simulink model "complex_fir_core"  (R2013a)
settings: Solver=VariableStepDiscrete  SolverMode=SingleTasking  StartTime=0.0  StopTime=2000  RelTol=1e-3
undefined symbols (not defined in the file or in its folder): pfb_coeff_gen_calc
libraries: xbsIndex_r4 x1618, casper_library_misc x112
(part 1 of 19)
settings Model: Creator=rprimian  LastModifiedBy=jack
settings Model: ModifiedComment=|
  | jack -- Wed Mar 18 10:34:12 2015 -- Version 1.45
  | resynth -lc off -equiv_reg_removal no
settings Model: ModifiedHistory=|
  | jack -- Wed Mar 18 10:34:12 2015 -- Version 1.45
  | resynth -lc off -equiv_reg_removal no
  | 
  | jack -- Wed Mar 18 10:28:24 2015 -- Version 1.44
  | change sync fanouter to have latency of 4 (max fanout 2)
  | 
  | jack -- Sun Jan 11 19:12:21 2015 -- Version 1.43
  | redrew with sync_delays implemented in srls when delay < 1024 (basically, always)
  | 
  | jack -- Sat Jan 10 15:01:06 2015 -- Version 1.42
  | generated
  | 
  | jack -- Sat Jan 10 13:10:56 2015 -- Version 1.41
  | update draw script to pipeline both fir cast blocks (was only pipelineing real one)
  | 
  | jack -- Fri Jan 09 11:30:49 2015 -- Version 1.40
  | 
  | 
  | jack -- Fri Jan 09 10:35:18 2015 -- Version 1.39
  | change add latency to 2. xlupdate model to 14.7
  | 
  | jack -- Fri Dec 05 12:22:04 2014 -- Version 1.38
  | compile test
  | 
  | cast latency3
settings DataIOCC: SignalLoggingSaveFormat=ModelDataLogs
settings OptimizationCC: InlineParams=on  ExpressionDepthLimit=2147483647
settings DebuggingCC: FcnCallInpInsideContextMsg=UseLocalSettings
settings GRTTargetCC: CombineOutputUpdateFcns=off  GRTInterface=on

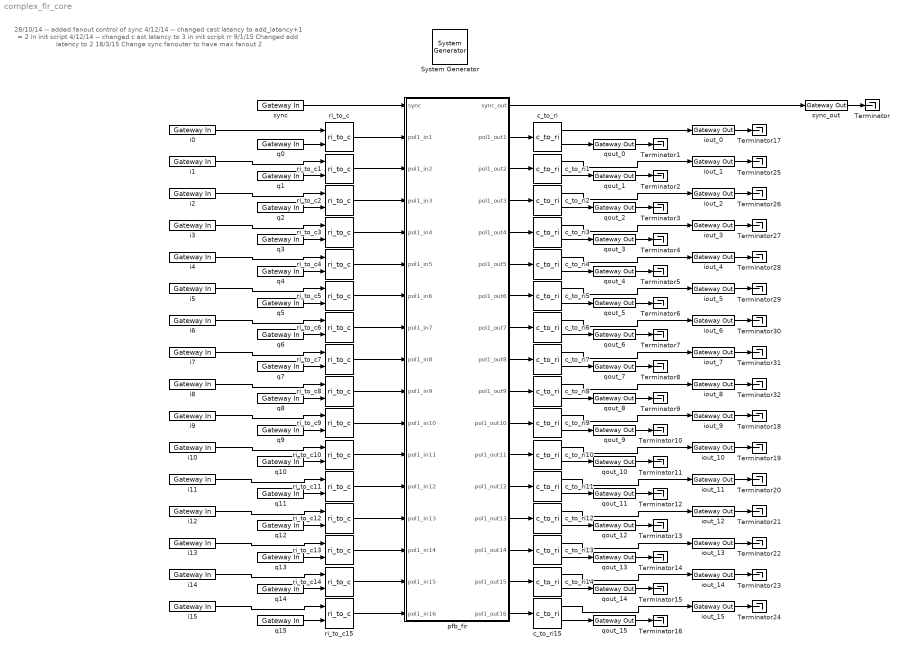
== system complex_fir_core ==
  note: 28/10/14 -- added fanout control of sync
      | 4/12/14 -- changed cast latency to add_latency+1 = 2 in init script
      | 4/12/14 -- changed c ast latency to 3 in init script rr
      | 9/1/15 Changed add latency to 2
      | 18/3/15 Change sync fanouter to have max fanout 2
  " System Generator" : xbsIndex_r4/ System Generator  Tag=genX  xilinxfamily=virtex6  part=xc6vsx475t  speed=-1  package=ff1759  synthesis_tool=XST  clock_wrapper=Clock Enables  directory=./complex_fir_core  proj_type=Project Navigator  Synth_file=XST Defaults  Impl_file=ISE Defaults  testbench=off  simulink_period=1  sysclk_period=3  dcm_input_clock_period=100  incr_netlist=off  trim_vbits=Everywhere in SubSystem  dbl_ovrd=According to Block Masks  core_generation=According to Block Masks  run_coregen=off  deprecated_control=off  eval_field=0  block_type=sysgen
      settings: block_version=11.4
  Terminator{,1..32} (33 alike) : Terminator
  c_to_ri{,1..15} (16 alike) : casper_library_misc/c_to_ri  n_bits=18  bin_pt=17
  i{0..15} (16 alike) : xbsIndex_r4/Gateway In  gui_display_data_type=Fixed-point  arith_type="Signed  (2's comp)"  n_bits=8  bin_pt=7  preci_type=Single  exp_width=8  frac_width=24  quantization="Round  (unbiased: +/- Inf)"  overflow=Saturate  period=1  dbl_ovrd=off  timing_constraint=None  locs_specified=off  LOCs={}  UseAsADC=off  ADCChannel='1'  inherit_from_input=off  hdl_port=on  block_type=gatewayin
      settings: infoedit="Gateway in block.  Converts inputs of type Simulink integer, double and fixed point to  Xilinx fixed point type.<br><br>Hardware notes:  In hardware these blocks become top level input ports."  block_version=11.4
  iout_{0..15} (16 alike) : xbsIndex_r4/Gateway Out  inherit_from_input=off  hdl_port=on  timing_constraint=None  locs_specified=off  LOCs={}  UseAsDAC=off  DACChannel='1'  block_type=gatewayout
      settings: infoedit="Gateway out block.  Converts Xilinx fixed point inputs into ouputs of type Simulink integer, double, or fixed point.<br><br>Hardware notes:  In hardware these blocks become top level output ports or are discarded, depending on how they are configured."  block_version=11.4
  pfb_fir : Subsystem  Tag=casper:pfb_fir  AncestorBlock=casper_library_pfbs/pfb_fir  mask(pfb_fir){PFBSize=12, TotalTaps=4, WindowType=hamming, n_inputs=4, MakeBiplex=off, BitWidthIn=8, BitWidthOut=18, CoeffBitWidth=18, CoeffDistMem=off, add_latency=2, mult_latency=3, bram_latency=3, fan_latency=1, quantization=Round  (unbiased: +/- Inf), fwidth=1, mult_spec=1, coeffs_share=on}
      mask prompts: PFBSize "Size of PFB: (2^? pnts)"; TotalTaps "Total Number of Taps:"; WindowType "Windowing Function:"; n_inputs "Number of Simultaneous Inputs: (2^?)"; MakeBiplex "Make Biplex?"; BitWidthIn "Input Bitwidth:"; BitWidthOut "Output Bitwidth:"; CoeffBitWidth "Coefficient Bitwidth:"; CoeffDistMem "Use Distributed Memory for Coeffs"; add_latency "Add Latency"; mult_latency "Mult Latency"; bram_latency "BRAM Latency"; fan_latency "Fanout Latency"; quantization "Quantization Behavior"; fwidth "Bin Width Scaling (normal=1)"; mult_spec "Multiplier specification (0=core, 1=embedded, 2=behavioural) (left=1st tap, or just one value)"; coeffs_share "Share coefficients between polarisations (use less BRAM)?"
      mask init:
      | pfb_fir_init(gcb, ...
      |     'PFBSize', PFBSize, ...
      |     'TotalTaps', TotalTaps, ...
      |     'WindowType', WindowType, ...
      |     'n_inputs', n_inputs, ...
      |     'MakeBiplex', MakeBiplex, ...
      |     'BitWidthIn', BitWidthIn, ...
      |     'BitWidthOut', BitWidthOut, ...
      |     'CoeffBitWidth', CoeffBitWidth, ...
      |     'CoeffDistMem', CoeffDistMem, ...
      |     'add_latency', add_latency, ...
      |     'mult_latency', mult_latency, ...
      |     'bram_latency', bram_latency, ...
      |     'fan_latency', fan_latency, ...
      |     'quantization', quantization, ...
      |     'fwidth', fwidth, ...
      |     'mult_spec', mult_spec, ...
      |     'coeffs_share', coeffs_share);
      settings: AttributesFormatString=|
      | taps=4, add_latency=2
      | max scale 0.596
      mask Help: eval('xlWeb(''http://casper.berkeley.edu/wiki/Pfb_fir'')')
      mask Callback TotalTaps:
      | %num_taps = eval(get_param(gcb, 'TotalTaps'));
      | %old_vec = eval(get_param(gcb, 'mult_spec'));
      | 
      | %vec = 2.*ones(1,num_taps);
      | %old_size = length(old_vec);
      | 
      | %if(old_size <= num_taps),
      | %   new_size = old_size;
      | %else,
      | %    new_size = num_taps;
      | %end
      | 
      | %for n = 1:new_size, vec(n) = old_vec(n); end
      | %set_param(gcb, 'mult_spec', mat2str(vec));
      mask TypeOptions WindowType: bartlett | barthannwin | blackman | blackmanharris | bohamwin | chebwin | flattopwin | gausswin | hamming | hann | kaiser | nuttallwin | parzenwin | rectwin | tukeywin | triang | userwindow
      mask TypeOptions quantization: Truncate | Round  (unbiased: +/- Inf) | Round  (unbiased: Even Values)
      mask Callback fwidth:
      | %num_taps = eval(get_param(gcb, 'TotalTaps'));
      | %old_vec = eval(get_param(gcb, 'mult_spec'));
      | 
      | %vec = 2.*ones(1,num_taps);
      | %old_size = length(old_vec);
      | 
      | %if(old_size <= num_taps),
      | %    new_size = old_size;
      | %else,
      | %    new_size = num_taps;
      | %end
      | 
      | %for n = 1:new_size, vec(n) = old_vec(n); end
      | %set_param(gcb, 'mult_spec', mat2str(vec));
      mask Callback mult_spec:
      | %num_taps = eval(get_param(gcb, 'TotalTaps'));
      | %old_vec = eval(get_param(gcb, 'mult_spec'));
      | 
      | %vec = 2.*ones(1,num_taps);
      | %old_size = length(old_vec);
      | 
      | %if(old_size <= num_taps),
      | %    new_size = old_size;
      | %else,
      | %    new_size = num_taps;
      | %end
      | 
      | %for n = 1:new_size, vec(n) = old_vec(n); end
      | %set_param(gcb, 'mult_spec', mat2str(vec));
  q{0..15} (16 alike) : xbsIndex_r4/Gateway In  gui_display_data_type=Fixed-point  arith_type="Signed  (2's comp)"  n_bits=8  bin_pt=7  preci_type=Single  exp_width=8  frac_width=24  quantization="Round  (unbiased: +/- Inf)"  overflow=Saturate  period=1  dbl_ovrd=off  timing_constraint=None  locs_specified=off  LOCs={}  UseAsADC=off  ADCChannel='1'  inherit_from_input=off  hdl_port=on  block_type=gatewayin
      settings: infoedit="Gateway in block.  Converts inputs of type Simulink integer, double and fixed point to  Xilinx fixed point type.<br><br>Hardware notes:  In hardware these blocks become top level input ports."  block_version=11.4
  qout_{0..15} (16 alike) : xbsIndex_r4/Gateway Out  inherit_from_input=off  hdl_port=on  timing_constraint=None  locs_specified=off  LOCs={}  UseAsDAC=off  DACChannel='1'  block_type=gatewayout
      settings: infoedit="Gateway out block.  Converts Xilinx fixed point inputs into ouputs of type Simulink integer, double, or fixed point.<br><br>Hardware notes:  In hardware these blocks become top level output ports or are discarded, depending on how they are configured."  block_version=11.4
  ri_to_c{,1..15} (16 alike) : casper_library_misc/ri_to_c
  sync : xbsIndex_r4/Gateway In  gui_display_data_type=Fixed-point  arith_type=Boolean  n_bits=1  bin_pt=0  preci_type=Single  exp_width=8  frac_width=24  quantization="Round  (unbiased: +/- Inf)"  overflow=Saturate  period=1  dbl_ovrd=off  timing_constraint=None  locs_specified=off  LOCs={}  UseAsADC=off  ADCChannel='1'  inherit_from_input=off  hdl_port=on  block_type=gatewayin
      settings: infoedit="Gateway in block.  Converts inputs of type Simulink integer, double and fixed point to  Xilinx fixed point type.<br><br>Hardware notes:  In hardware these blocks become top level input ports."  block_version=11.4
  sync_out : xbsIndex_r4/Gateway Out  inherit_from_input=off  hdl_port=on  timing_constraint=None  locs_specified=off  LOCs={}  UseAsDAC=off  DACChannel='1'  block_type=gatewayout
      settings: infoedit="Gateway out block.  Converts Xilinx fixed point inputs into ouputs of type Simulink integer, double, or fixed point.<br><br>Hardware notes:  In hardware these blocks become top level output ports or are discarded, depending on how they are configured."  block_version=11.4
  wires:
  sync_out/1 -> Terminator/1
  qout_0/1 -> Terminator1/1
  qout_1/1 -> Terminator2/1
  qout_2/1 -> Terminator3/1
  qout_3/1 -> Terminator4/1
  qout_4/1 -> Terminator5/1
  qout_5/1 -> Terminator6/1
  qout_6/1 -> Terminator7/1
  qout_7/1 -> Terminator8/1
  qout_8/1 -> Terminator9/1
  qout_9/1 -> Terminator10/1
  qout_10/1 -> Terminator11/1
  qout_11/1 -> Terminator12/1
  qout_12/1 -> Terminator13/1
  qout_13/1 -> Terminator14/1
  qout_14/1 -> Terminator15/1
  qout_15/1 -> Terminator16/1
  ri_to_c/1 -> pfb_fir/2(pol1_in1)
  ri_to_c1/1 -> pfb_fir/3(pol1_in2)
  sync/1 -> pfb_fir/1(sync)
  ri_to_c2/1 -> pfb_fir/4(pol1_in3)
  ri_to_c3/1 -> pfb_fir/5(pol1_in4)
  ri_to_c5/1 -> pfb_fir/7(pol1_in6)
  ri_to_c4/1 -> pfb_fir/6(pol1_in5)
  ri_to_c7/1 -> pfb_fir/9(pol1_in8)
  ri_to_c6/1 -> pfb_fir/8(pol1_in7)
  ri_to_c10/1 -> pfb_fir/12(pol1_in11)
  ri_to_c9/1 -> pfb_fir/11(pol1_in10)
  ri_to_c13/1 -> pfb_fir/15(pol1_in14)
  ri_to_c12/1 -> pfb_fir/14(pol1_in13)
  ri_to_c8/1 -> pfb_fir/10(pol1_in9)
  ri_to_c14/1 -> pfb_fir/16(pol1_in15)
  ri_to_c15/1 -> pfb_fir/17(pol1_in16)
  ri_to_c11/1 -> pfb_fir/13(pol1_in12)
  pfb_fir/1(sync_out) -> sync_out/1
  pfb_fir/2(pol1_out1) -> c_to_ri/1
  pfb_fir/3(pol1_out2) -> c_to_ri1/1
  pfb_fir/4(pol1_out3) -> c_to_ri2/1
  pfb_fir/5(pol1_out4) -> c_to_ri3/1
  pfb_fir/6(pol1_out5) -> c_to_ri4/1
  pfb_fir/7(pol1_out6) -> c_to_ri5/1
  pfb_fir/8(pol1_out7) -> c_to_ri6/1
  pfb_fir/9(pol1_out8) -> c_to_ri7/1
  pfb_fir/10(pol1_out9) -> c_to_ri8/1
  pfb_fir/11(pol1_out10) -> c_to_ri9/1
  pfb_fir/12(pol1_out11) -> c_to_ri10/1
  pfb_fir/13(pol1_out12) -> c_to_ri11/1
  pfb_fir/14(pol1_out13) -> c_to_ri12/1
  pfb_fir/15(pol1_out14) -> c_to_ri13/1
  pfb_fir/16(pol1_out15) -> c_to_ri14/1
  pfb_fir/17(pol1_out16) -> c_to_ri15/1
  i0/1 -> ri_to_c/1
  i1/1 -> ri_to_c1/1
  i2/1 -> ri_to_c2/1
  i3/1 -> ri_to_c3/1
  i4/1 -> ri_to_c4/1
  i5/1 -> ri_to_c5/1
  i6/1 -> ri_to_c6/1
  i7/1 -> ri_to_c7/1
  i8/1 -> ri_to_c8/1
  i9/1 -> ri_to_c9/1
  i10/1 -> ri_to_c10/1
  i11/1 -> ri_to_c11/1
  i12/1 -> ri_to_c12/1
  i13/1 -> ri_to_c13/1
  i14/1 -> ri_to_c14/1
  i15/1 -> ri_to_c15/1
  q0/1 -> ri_to_c/2
  q1/1 -> ri_to_c1/2
  q2/1 -> ri_to_c2/2
  q3/1 -> ri_to_c3/2
  q4/1 -> ri_to_c4/2
  q5/1 -> ri_to_c5/2
  q6/1 -> ri_to_c6/2
  q7/1 -> ri_to_c7/2
  q8/1 -> ri_to_c8/2
  q9/1 -> ri_to_c9/2
  q10/1 -> ri_to_c10/2
  q11/1 -> ri_to_c11/2
  q12/1 -> ri_to_c12/2
  q13/1 -> ri_to_c13/2
  q14/1 -> ri_to_c14/2
  q15/1 -> ri_to_c15/2
  iout_0/1 -> Terminator17/1
  iout_1/1 -> Terminator25/1
  iout_2/1 -> Terminator26/1
  iout_3/1 -> Terminator27/1
  iout_4/1 -> Terminator28/1
  iout_5/1 -> Terminator29/1
  iout_6/1 -> Terminator30/1
  iout_7/1 -> Terminator31/1
  iout_8/1 -> Terminator32/1
  iout_9/1 -> Terminator18/1
  iout_10/1 -> Terminator19/1
  iout_11/1 -> Terminator20/1
  iout_12/1 -> Terminator21/1
  iout_13/1 -> Terminator22/1
  iout_14/1 -> Terminator23/1
  iout_15/1 -> Terminator24/1
  c_to_ri/1 -> iout_0/1
  c_to_ri/2 -> qout_0/1
  c_to_ri1/1 -> iout_1/1
  c_to_ri1/2 -> qout_1/1
  c_to_ri2/1 -> iout_2/1
  c_to_ri2/2 -> qout_2/1
  c_to_ri3/1 -> iout_3/1
  c_to_ri3/2 -> qout_3/1
  c_to_ri4/1 -> iout_4/1
  c_to_ri4/2 -> qout_4/1
  c_to_ri5/1 -> iout_5/1
  c_to_ri5/2 -> qout_5/1
  c_to_ri6/1 -> iout_6/1
  c_to_ri6/2 -> qout_6/1
  c_to_ri7/1 -> iout_7/1
  c_to_ri7/2 -> qout_7/1
  c_to_ri8/1 -> iout_8/1
  c_to_ri8/2 -> qout_8/1
  c_to_ri9/1 -> iout_9/1
  c_to_ri9/2 -> qout_9/1
  c_to_ri10/1 -> iout_10/1
  c_to_ri10/2 -> qout_10/1
  c_to_ri11/1 -> iout_11/1
  c_to_ri11/2 -> qout_11/1
  c_to_ri12/1 -> iout_12/1
  c_to_ri12/2 -> qout_12/1
  c_to_ri13/1 -> iout_13/1
  c_to_ri13/2 -> qout_13/1
  c_to_ri14/1 -> iout_14/1
  c_to_ri14/2 -> qout_14/1
  c_to_ri15/1 -> iout_15/1
  c_to_ri15/2 -> qout_15/1
